simulink model "exercise3Simu"  (R2020b)
settings: Solver=VariableStepAuto  StartTime=0.0  StopTime=20  RelTol=1e-3
values from neighbouring files (symbols this model uses):
  CD = -2    [exercise1.m]
  gc = -32.2    [exercise1.m]
  m = mlbm/gc    (= -3.16770186335)    [exercise1.m]
settings Model: Creator=mreiff  LastModifiedBy=mreiff

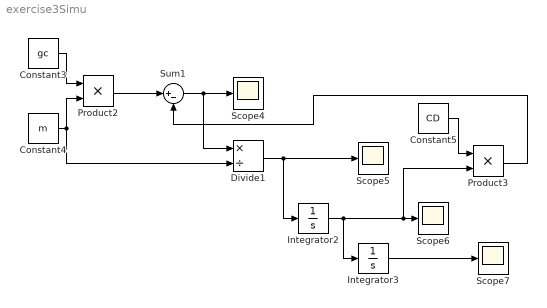
== system exercise3Simu ==
  Constant3 : Constant  Value=gc
  Constant4 : Constant  Value=m
  Constant5 : Constant  Value=CD
  Divide1 : Product  Inputs=*/
  Integrator2 : Integrator  InitialCondition=200
  Integrator3 : Integrator  InitialCondition=10
  Product2 : Product
  Product3 : Product
  Scope{4..7} (4 alike) : Scope
  Sum1 : Sum  Inputs=|+-
  wires:
  Constant3/1 -> Product2/1
  Constant4/1 -> Divide1/2, Product2/2
  Product2/1 -> Sum1/1
  Sum1/1 -> Divide1/1, Scope4/1
  Divide1/1 -> Integrator2/1, Scope5/1
  Integrator2/1 -> Integrator3/1, Product3/2, Scope6/1
  Integrator3/1 -> Scope7/1
  Constant5/1 -> Product3/1
  Product3/1 -> Sum1/2
